simulink model "Fuzzy PID Controller"  (R2020b)
settings: Solver=VariableStepAuto  StartTime=0.0  StopTime=500  RelTol=1e-3
model workspace (MAT data in the model file):
  InS = 30
undefined symbols (not defined in the file): A, B, C, D
libraries: simulink x1, fuzblock x1
settings Model: Creator=rohan  LastModifiedBy=rohan

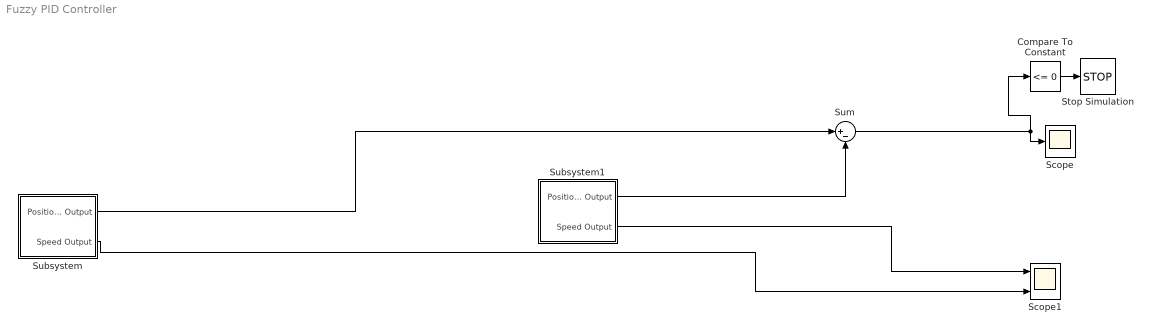
== system Fuzzy PID Controller ==
  Compare To Constant : simulink/Logic and Bit Operations/Compare To Constant  relop=<=  const=0  OutDataTypeStr=boolean
  Scope : Scope
  Scope1 : Scope  NumInputPorts=2
  Stop Simulation : Stop
  Subsystem : Subsystem
  Subsystem1 : Subsystem
  Sum : Sum  Inputs=|+-
  wires:
  Compare To Constant/1 -> Stop Simulation/1
  Sum/1 -> Scope/1, Compare To Constant/1
  Subsystem/1(Position Output) -> Sum/1
  Subsystem1/1(Position Output) -> Sum/2
  Subsystem/2(Speed Output) -> Scope1/2
  Subsystem1/2(Speed Output) -> Scope1/1

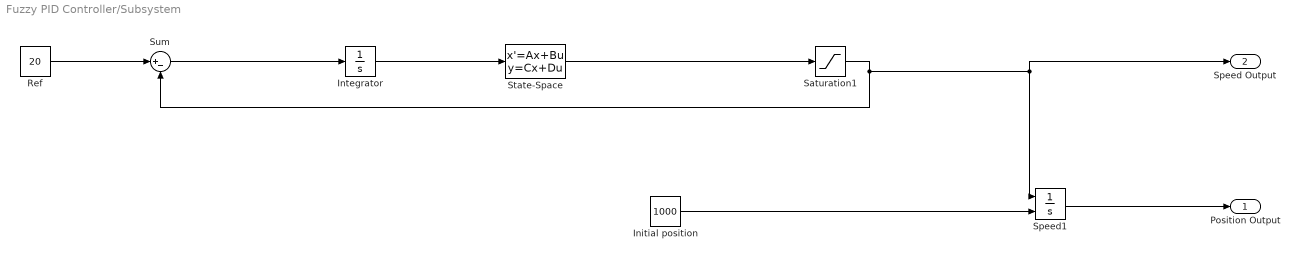
== system Fuzzy PID Controller/Subsystem ==
  Initial position : Constant  Value=1000
  Integrator : Integrator
  Ref : Constant  Value=20
  Saturation1 : Saturate  UpperLimit=40  LowerLimit=0
  Speed1 : Integrator  InitialConditionSource=external
  State-Space : StateSpace  A=A  B=B  C=C  D=D  InitialCondition=25
  Sum : Sum  Inputs=|+-
  Position Output : Outport
  Speed Output : Outport  Port=2
  wires:
  Sum/1 -> Integrator/1
  Ref/1 -> Sum/1
  Saturation1/1 -> Sum/2, Speed Output/1, Speed1/1
  Initial position/1 -> Speed1/2
  Speed1/1 -> Position Output/1
  State-Space/1 -> Saturation1/1
  Integrator/1 -> State-Space/1

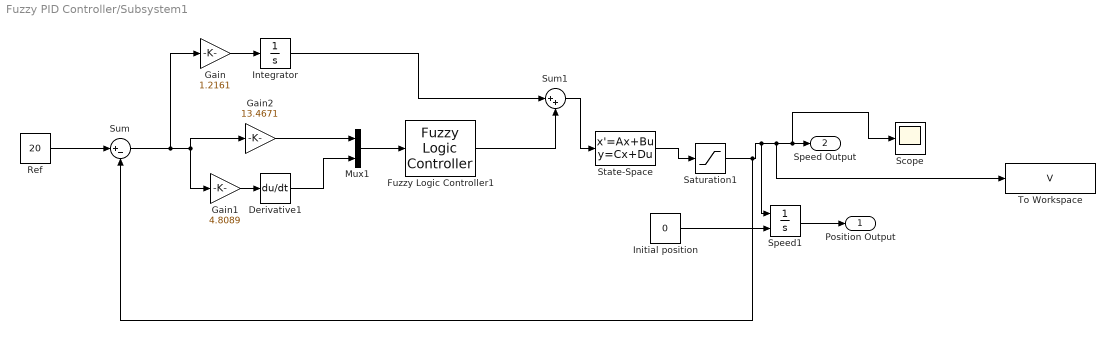
== system Fuzzy PID Controller/Subsystem1 ==
  Derivative1 : Derivative
  Fuzzy Logic Controller1 : fuzblock/Fuzzy Logic  Controller  FIS=abc1  OutputSampleNumber=101  DataType=double  FuzzifiedInputs=off  RuleFiringStrengths=off  RuleOutputs=off  AggregatedOutputs=off  SimulateUsing=Interpreted execution  OutOfRangeInputValueMessage=warning  NoRuleFiredMessage=warning  EmptyOutputFuzzySetMessage=warning
  Gain : Gain  Gain=1.2161
  Gain1 : Gain  Gain=4.8089
  Gain2 : Gain  Gain=13.4671
  Initial position : Constant  Value=0
  Integrator : Integrator
  Mux1 : Mux  Inputs=2
  Ref : Constant  Value=20
  Saturation1 : Saturate  UpperLimit=100  LowerLimit=0
  Scope : Scope
  Speed1 : Integrator  InitialConditionSource=external
  State-Space : StateSpace  A=A  B=B  C=C  D=0  InitialCondition=40
  Sum : Sum  Inputs=|+-
  Sum1 : Sum  Inputs=|++
  To Workspace : ToWorkspace  VariableName=V  SaveFormat=Timeseries  SampleTime=1
  Position Output : Outport
  Speed Output : Outport  Port=2
  wires:
  Saturation1/1 -> Sum/2, To Workspace/1, Scope/1, Speed Output/1, Speed1/1
  Initial position/1 -> Speed1/2
  Speed1/1 -> Position Output/1
  State-Space/1 -> Saturation1/1
  Derivative1/1 -> Mux1/2
  Mux1/1 -> Fuzzy Logic Controller1/1
  Ref/1 -> Sum/1
  Integrator/1 -> Sum1/1
  Fuzzy Logic Controller1/1 -> Sum1/2
  Sum1/1 -> State-Space/1
  Sum/1 -> Gain/1, Gain1/1, Gain2/1
  Gain/1 -> Integrator/1
  Gain2/1 -> Mux1/1
  Gain1/1 -> Derivative1/1
